simulink model "untitled"  (R2018b)
settings: Solver=VariableStepAuto  StartTime=0.0  StopTime=200  RelTol=1e-3
values from neighbouring files (symbols this model uses):
  R = [1 X(1)]    [pruebaloDePagina.m]
  S = X(2:end)'    [pruebaloDePagina.m]
undefined symbols (not defined in the file or in its folder): M1D
settings Model: Creator=AlfredoMaussa  LastModifiedBy=AlfredoMaussa

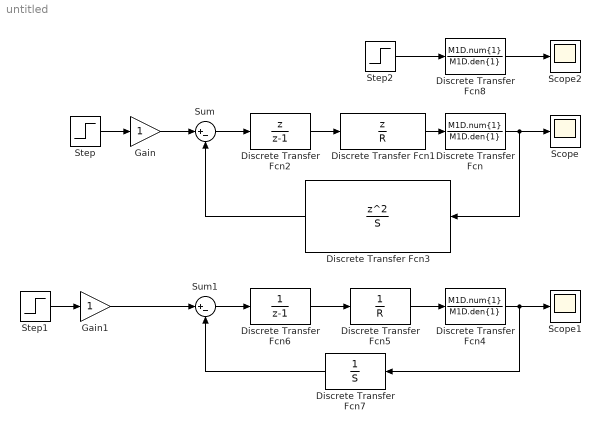
== system untitled ==
  Discrete Transfer Fcn : DiscreteTransferFcn  Numerator=M1D.num{1}  Denominator=M1D.den{1}
  Discrete Transfer Fcn1 : DiscreteTransferFcn  Numerator=[1,0]  Denominator=R  SampleTime=0.005
  Discrete Transfer Fcn2 : DiscreteTransferFcn  Numerator=[1,0]  Denominator=[1,-1]
  Discrete Transfer Fcn3 : DiscreteTransferFcn  Numerator=[1,0,0]  Denominator=S
  Discrete Transfer Fcn4 : DiscreteTransferFcn  Numerator=M1D.num{1}  Denominator=M1D.den{1}  SampleTime=0.005
  Discrete Transfer Fcn5 : DiscreteTransferFcn  Numerator=1  Denominator=R
  Discrete Transfer Fcn6 : DiscreteTransferFcn  Numerator=1  Denominator=[1,-1]  SampleTime=0.005
  Discrete Transfer Fcn7 : DiscreteTransferFcn  Numerator=1  Denominator=S
  Discrete Transfer Fcn8 : DiscreteTransferFcn  Numerator=M1D.num{1}  Denominator=M1D.den{1}
  Gain : Gain
  Gain1 : Gain
  Scope : Scope
  Scope1 : Scope
  Scope2 : Scope
  Step : Step  Time=0  SampleTime=0
  Step1 : Step  Time=0  SampleTime=0
  Step2 : Step  Time=0  SampleTime=0
  Sum : Sum  Inputs=|+-
  Sum1 : Sum  Inputs=|+-
  wires:
  Discrete Transfer Fcn1/1 -> Discrete Transfer Fcn/1
  Discrete Transfer Fcn2/1 -> Discrete Transfer Fcn1/1
  Sum/1 -> Discrete Transfer Fcn2/1
  Discrete Transfer Fcn/1 -> Scope/1, Discrete Transfer Fcn3/1
  Gain/1 -> Sum/1
  Step/1 -> Gain/1
  Step1/1 -> Gain1/1
  Gain1/1 -> Sum1/1
  Discrete Transfer Fcn7/1 -> Sum1/2
  Discrete Transfer Fcn4/1 -> Discrete Transfer Fcn7/1, Scope1/1
  Sum1/1 -> Discrete Transfer Fcn6/1
  Discrete Transfer Fcn6/1 -> Discrete Transfer Fcn5/1
  Discrete Transfer Fcn5/1 -> Discrete Transfer Fcn4/1
  Step2/1 -> Discrete Transfer Fcn8/1
  Discrete Transfer Fcn8/1 -> Scope2/1
  Discrete Transfer Fcn3/1 -> Sum/2
